simulink model "dwupolozeniowy_kor"  (R2018b)
settings: Solver=VariableStepAuto  StartTime=0.0  StopTime=100  RelTol=1e-3
settings Model: Creator=groinder  LastModifiedBy=krzys

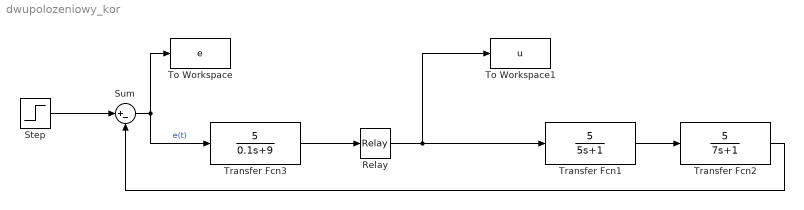
== system dwupolozeniowy_kor ==
  Relay : Relay  OnSwitchValue=0  OffSwitchValue=0
  Step : Step  SampleTime=0
  Sum : Sum  Inputs=|+-
  To Workspace : ToWorkspace  VariableName=e  SaveFormat=Structure With Time  SampleTime=-1
  To Workspace1 : ToWorkspace  VariableName=u  SaveFormat=Structure With Time  SampleTime=-1
  Transfer Fcn1 : TransferFcn  Numerator=[5]  Denominator=[5 1]
  Transfer Fcn2 : TransferFcn  Numerator=[5]  Denominator=[7 1]
  Transfer Fcn3 : TransferFcn  Numerator=[5]  Denominator=[0.1 9]
  wires:
  Step/1 -> Sum/1
  Sum/1 -> To Workspace/1, Transfer Fcn3/1  "e(t)"
  Transfer Fcn1/1 -> Transfer Fcn2/1
  Relay/1 -> Transfer Fcn1/1, To Workspace1/1
  Transfer Fcn3/1 -> Relay/1
  Transfer Fcn2/1 -> Sum/2
